simulink model "ControlFuzzyPendulo"  (Simulink 8.9)
settings: Solver=ode45  StartTime=0.0  StopTime=40  RelTol=1e-3  EnableMultiTasking=on
libraries: fuzblock x1
settings Model: Creator=yo  LastModifiedBy=Dell  ExtModeTrigMode=oneshot  ExtModeArmWhenConnect=off
settings SolverCC: ZeroCrossControl=DisableAll
settings DataIOCC: LimitDataPoints=off  SignalLoggingName=sigsOut
settings OptimizationCC: BlockReduction=off  BooleanDataType=off  ExpressionDepthLimit=2147483647  InitFltsAndDblsToZero=on
settings DebuggingCC: SaveWithParameterizedLinksMsg=none  SignalResolutionControl=TryResolveAllWithWarning  MultiTaskDSMMsg=warning  MultiTaskCondExecSysMsg=none
settings HardwareCC: TargetUnknown=on
settings GRTTargetCC: GeneratePreprocessorConditionals=Use local settings

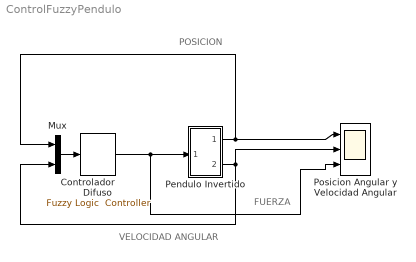
== system ControlFuzzyPendulo ==
  note: POSICION
  note: VELOCIDAD ANGULAR
  note: FUERZA
  "   Controlador        Difuso" : fuzblock/Fuzzy Logic  Controller  fis=readfis('sugeno_pendulum.fis')
  " Pendulo Invertido" : Subsystem  mask(Cart & Pole){init_cond=[0.4, 0, 0, 0], specs=[0.5, 0.1, 1.0, 9.8]}
      mask prompts: init_cond "Initial Conditions (angle, angular velocity, cart position and cart velocity):"; specs "Physical Specifications (pole length, pole mass, cart mass and g):"
      mask help: Inverted Pendulum (cart & pole)
      mask init:
      | l=specs(1)/2;m=specs(2);mc=specs(3);g=specs(4);
      mask Help: Inverted Pendulum
      mask Display: plot(-4,-1,4,6,[0 3 2.8 -0.2 0],[1 5 5.15 1.15 1],[-1 -1 1 1 -1],[1 0 0 1 1],[-3.5 3.5],[0 0])
  Mux : Mux  Inputs=2
  Posicion Angular y Velocidad Angular : Scope  NumInputPorts=3
  wires:
  " Pendulo Invertido"/1(out_1) -> Mux/1, Posicion Angular y Velocidad Angular/1
  "   Controlador        Difuso"/1 -> Posicion Angular y Velocidad Angular/3, " Pendulo Invertido"/1(in_1)
  Mux/1 -> "   Controlador        Difuso"/1
  " Pendulo Invertido"/2(out_2) -> Mux/2, Posicion Angular y Velocidad Angular/2

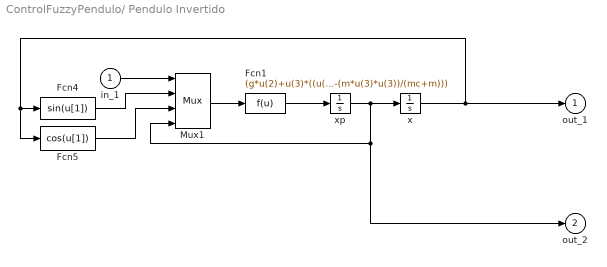
== system ControlFuzzyPendulo/ Pendulo Invertido ==
  in_1 : Inport
  Fcn1 : Fcn  Expr=(g*u(2)+u(3)*((u(1)-m*l*u(4)*u(4)*u(2))/(mc+m)))/(l*(4/3-(m*u(3)*u(3))/(mc+m)))
  Fcn4 : Fcn
  Fcn5 : Fcn  Expr=cos(u[1])
  Mux1 : Mux
  x : Integrator  InitialCondition=init_cond(1)
  xp : Integrator  InitialCondition=init_cond(2)
  out_1 : Outport  InitialOutput=0
  out_2 : Outport  Port=2  InitialOutput=0
  wires:
  in_1/1 -> Mux1/1
  xp/1 -> x/1, Mux1/4, out_2/1
  Fcn4/1 -> Mux1/2
  Fcn5/1 -> Mux1/3
  x/1 -> Fcn4/1, Fcn5/1, out_1/1
  Mux1/1 -> Fcn1/1
  Fcn1/1 -> xp/1
